simulink model "SPWM_5_Level"  (R2014a)
settings: Solver=ode45  StartTime=0.0  StopTime=0.06  RelTol=1e-3
libraries: powerlib x14, simulink x4
settings Model: Creator=RAVINDERNATH YADAV  LastModifiedBy=RAVINDERNATH YADAV

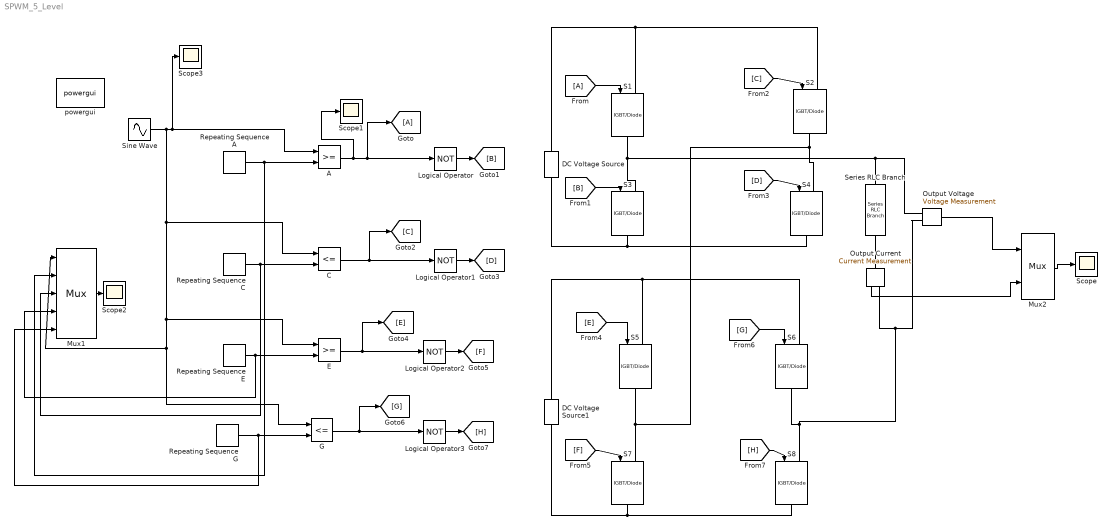
== system SPWM_5_Level ==
  "A " : RelationalOperator  OutDataTypeStr=boolean
  "C " : RelationalOperator  Operator=<=  OutDataTypeStr=boolean
  DC Voltage Source : powerlib/Electrical Sources/DC Voltage Source  Amplitude=2  Measurements=None
  DC Voltage Source1 : powerlib/Electrical Sources/DC Voltage Source  Amplitude=2  Measurements=None
  E : RelationalOperator  OutDataTypeStr=boolean
  G : RelationalOperator  Operator=<=  OutDataTypeStr=boolean
  Logical Operator{,1..3} (4 alike) : Logic  Operator=NOT  AllPortsSameDT=off  OutDataTypeStr=boolean
  Mux1 : Mux  Inputs=5
  Mux2 : Mux  Inputs=2
  Output Current : powerlib/Measurements/Current Measurement  PhasorSimulation=off  OutputType=Complex  PSBequivalent=0
  "Output Voltage " : powerlib/Measurements/Voltage Measurement  PhasorSimulation=off  OutputType=Complex  PSBequivalent=0
  Repeating Sequence A : simulink/Sources/Repeating Sequence  rep_seq_t=[0 0.5 1]/(21*50)  rep_seq_y=[0.5 1 0.5]
  Repeating Sequence C : simulink/Sources/Repeating Sequence  rep_seq_t=[0 0.5 1]/(21*50)  rep_seq_y=[0 0.5 0]
  Repeating Sequence E : simulink/Sources/Repeating Sequence  rep_seq_t=[0 0.5 1]/(21*50)  rep_seq_y=[-0.5 0 -0.5]
  "Repeating Sequence G " : simulink/Sources/Repeating Sequence  rep_seq_t=[0 0.5 1]/(21*50)  rep_seq_y=[-1 -0.5 -1]
  S{1..8} (8 alike) : powerlib/Power Electronics/IGBT//Diode  Ron=1e-3  Rs=1e5  Cs=inf  Measurements=off
  Scope{,1..3} (4 alike) : Scope
      Scope settings: ShowLegends=on  TimeRange=0.02  YMin=-6  YMax=6
      Scope1 settings: ShowLegends=on  TimeRange=0.1  YMin=-1  YMax=1.5
      Scope2 settings: ShowLegends=on  TimeRange=0.1  YMin=-1  YMax=1.5  SaveName=ScopeData2
      Scope3 settings: ShowLegends=on  TimeRange=0.1  YMin=-1  YMax=1.5  SaveName=ScopeData3
  Series RLC Branch : powerlib/Elements/Series RLC Branch  LConnTagsString=__new0  RConnTagsString=__new0  BranchType=R  Resistance=10  Inductance=1e-3  SetiL0=off  InitialCurrent=0  Capacitance=1e-6  Setx0=off  InitialVoltage=0  Measurements=None
  Sine Wave : Sin  Frequency=2*3.14*50  SampleTime=0
  powergui : powerlib/powergui  Priority=1  SimulationMode=Discrete  SolverType=Tustin  SampleTime=50e-6  frequency=60  SPID=off  DisableSnubberDevices=off  DisableRonSwitches=off  DisableVfSwitches=off  SwTol=0  Interpol=off  DisplayEquations=off  Ts=0  methode=off  frequencyindice=0  Pbase=100e6  ErrMax=1e-4  Iterations=50  UnitsV=kV  UnitsW=MW  FunctionMessages=off  echomessages=off  HookPort=off  EnableUseOfTLC=off  x0status=blocks  RestoreLinks=warning  ResistiveCurrentMeasurement=off  Frange=[0:2:500]  Ylog=off  Xlog=on  ShowGrid=off  save=off  variable=ZData  structure=logsout  ZoomFFT=off  StartTime=0.0  cycles=1  DisplayStyle=1  fundamental=50  FreqAxis=off  MaxFrequency=1000  frequencyindicesteady=1  RmsSteady=1  display=off
  wires:
  Repeating Sequence A/1 -> Mux1/2, "A "/2
  Repeating Sequence C/1 -> Mux1/3, "C "/2
  "C "/1 -> [C], Logical Operator1/1
  Repeating Sequence E/1 -> E/2, Mux1/4
  E/1 -> [E], Logical Operator2/1
  "Repeating Sequence G "/1 -> Mux1/5, G/2
  G/1 -> [G], Logical Operator3/1
  Mux1/1 -> Scope2/1
  Sine Wave/1 -> Mux1/1, G/1, E/1, "C "/1, Scope3/1, "A "/1
  Logical Operator/1 -> [B]
  Logical Operator1/1 -> [D]
  Logical Operator2/1 -> [F]
  "A "/1 -> Scope1/1, [A], Logical Operator/1
  [A] -> S1/1
  [B] -> S3/1
  [C] -> S2/1
  [D] -> S4/1
  [E] -> S5/1
  [F] -> S7/1
  [G] -> S6/1
  Logical Operator3/1 -> [H]
  [H] -> S8/1
  Mux2/1 -> Scope/1
  "Output Voltage "/1 -> Mux2/1
  Output Current/1 -> Mux2/2
  connections:
  DC Voltage Source/LConn1 -- S4/RConn1 -- S3/RConn1
  S1/LConn1 -- S2/LConn1 -- DC Voltage Source/RConn1
  S6/LConn1 -- DC Voltage Source1/RConn1 -- S5/LConn1
  S7/RConn1 -- S8/RConn1 -- DC Voltage Source1/LConn1
  Output Current/RConn1 -- S6/RConn1 -- S8/LConn1 -- "Output Voltage "/LConn2
  Series RLC Branch/RConn1 -- Output Current/LConn1
  S1/RConn1 -- "Output Voltage "/LConn1 -- Series RLC Branch/LConn1 -- S3/LConn1
  S2/RConn1 -- S7/LConn1 -- S5/RConn1 -- S4/LConn1
